simulink model "Task6"  (R2024a)
settings: Solver=VariableStepAuto  StartTime=0.0  StopTime=100.0  RelTol=1e-3
settings Model: Creator=artemzmailov  LastModifiedBy=artemzmailov

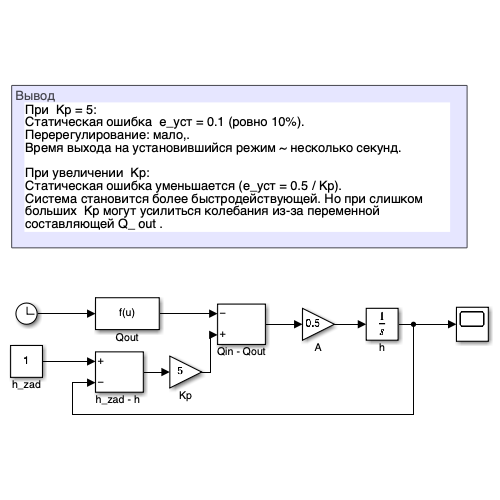
[thumbnail: Simulink's stored preview of the top-level diagram]
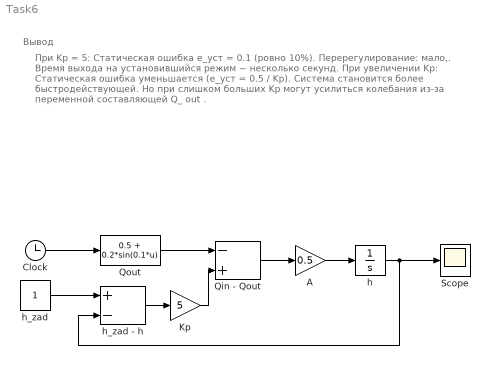
== system Task6 ==
  note: Вывод
  note: При Kp = 5:
      | Статическая ошибка e_уст = 0.1 (ровно 10%).
      | Перерегулирование: мало,.
      | Время выхода на установившийся режим ~ несколько секунд.
      |
      | При увеличении Kp:
      | Статическая ошибка уменьшается (e_уст = 0.5 / Kp).
      | Система становится более быстродействующей. Но при слишком больших Kp могут усилиться колебания из-за переменной составляющей Q_ out .
  A : Gain  Gain=0.5
  Clock : Clock
  Kp : Gain  Gain=5
  Qin - Qout : Sum  Inputs=-+
  Qout : Fcn  Expr=0.5 + 0.2*sin(0.1*u)
  Scope : Scope
  h : Integrator  InitialCondition=0.8
  h_zad : Constant
  "h_zad - h " : Sum  Inputs=+-
  wires:
  Clock/1 -> Qout/1
  Qout/1 -> Qin - Qout/1
  "h_zad - h "/1 -> Kp/1
  Kp/1 -> Qin - Qout/2
  h_zad/1 -> "h_zad - h "/1
  h/1 -> Scope/1, "h_zad - h "/2
  Qin - Qout/1 -> A/1
  A/1 -> h/1
